simulink model "test_plant"  (R2023a)
settings: Solver=ode5  StartTime=0.0  StopTime=96  FixedStep=1.0  RelTol=1e-3
undefined symbols (not defined in the file): Standard_Devices, UDP_Protocol
libraries: sldrtlib x3, embmathops x1
settings Model: Creator=The MathWorks, Inc.  LastModifiedBy=umphaipunatipunumphai
settings SolverCC: AlgebraicLoopSolver=TrustRegion  DecoupledContinuousIntegration=on  MinimalZcImpactIntegration=on
settings DataIOCC: ReturnWorkspaceOutputs=off
settings DebuggingCC: UnconnectedInputMsg=warning  UnconnectedOutputMsg=warning  UnconnectedLineMsg=warning  PregeneratedLibrarySubsystemCodeDiagnostic=none  ArithmeticOperatorsInVariantConditions=warning
settings HardwareCC: ProdBitPerLong=64  ProdHWDeviceType=Intel->x86-64 (Linux 64)
settings ModelReferenceCC: EnableRefExpFcnMdlSchedulingChecks=on
settings SFSimCC: SimUseLocalCustomCode=off  CustomCodeUndefinedFunction=UseInterfaceOnly
settings RTWCC: Description=Simulink Desktop Real-Time  SystemTargetFile=sldrt.tlc  TemplateMakefile=sldrt.tmf  RTWUseLocalCustomCode=off  RTWCompilerOptimization=on  DLArmComputeVersion=19.05
settings CodeAppCC: MaxIdLength=95
settings SimulinkDesktopRealTimeCC: TargetLibSuffix=_sldrt.a  TargetPreCompLibLocation=/Applications/MATLAB_R2023a.app/toolbox/sldrt/lib/maci64

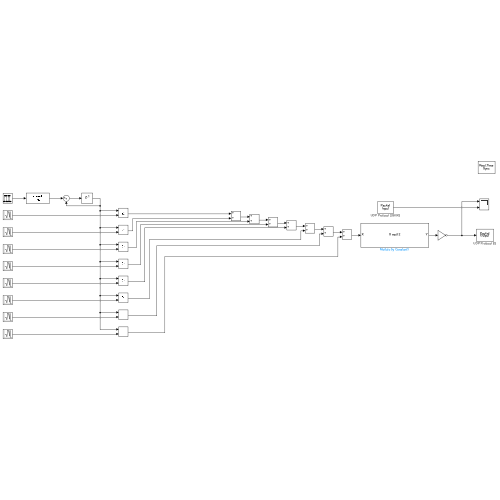
[thumbnail: Simulink's stored preview of the top-level diagram]
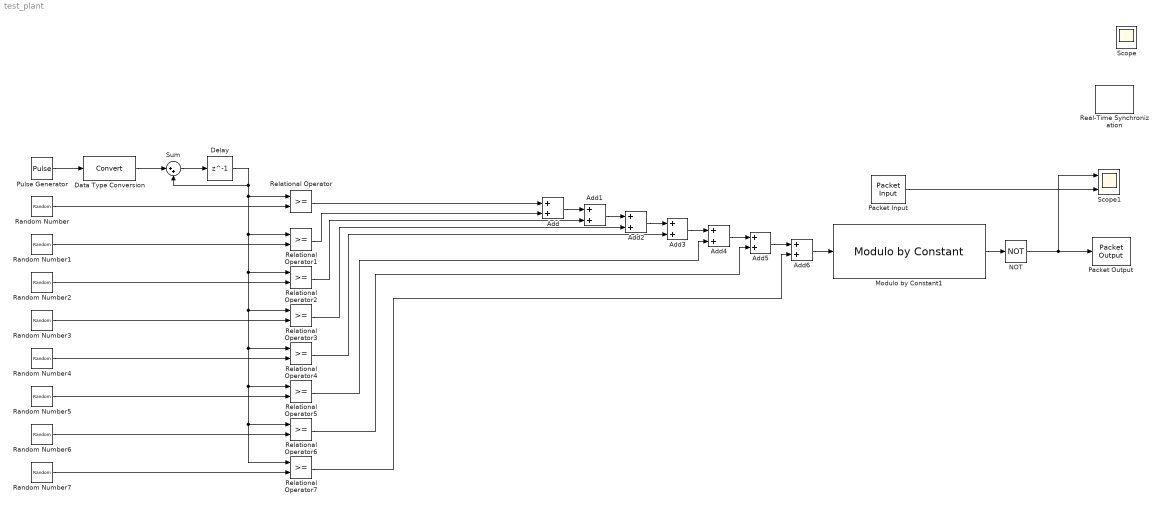
== system test_plant ==
  Add{,1..6} (7 alike) : Sum
  Data Type Conversion : DataTypeConversion  OutMin=0  OutMax=1  ConvertRealWorld=Stored Integer (SI)  RndMeth=Nearest  SaturateOnIntegerOverflow=off
  Delay : Delay  DelayLength=1  InitialCondition=0  SampleTime=1
  Modulo by Constant1 : embmathops/Modulo by Constant  Denominator=2  SimulateUsing=Code generation
      settings: LibrarySourceBlock=embeddedMathLib/Modulo by Constant
  NOT : Logic  Operator=NOT  IconShape=distinctive  AllPortsSameDT=off  OutDataTypeStr=boolean
  Packet Input : sldrtlib/Packet Input  SampleTime=1  MaxMissedTicks=10  ShowMissedTicks=off  YieldWhenWaiting=on  DrvName=Standard_Devices/UDP_Protocol  DrvAddress=26000  DrvOptions=[0 0 114 112 105 99 112 115 46 109 115 104 111 109 101 46 110 101 116 0 0 0 0 0 0 0 0 0 0 0 0 0 0 0 0 0 0 0 0 0 0 0 0 0 0 0 0 0 0 0 0 0 0 0 0 0 0 0 0 0 0 0 0 0 0 0 0 0 0 0 0 0 0 0 0 0 0 0 0 0 0 0 0 0 0 0 0 0 0 0 0 0 0 0 0 0 0 0 0 0 0 0 0 0 0 0 0 0 0 0 0 0 0 0 0 0 0 0 0 0 0 0 0 0 0 0 0 0 0 0 0 0 0 0 0 0 0 0 0 0 0 0 0 0 0 0 0 0 0 0 0 0 0 0 0 0 0 0 0 0 0 0 0 0 0 0 0 0 0 0 0 0 0 0 0 0 0 0 0 0 0 0 0 0 0 0 0 0 0 0 0 0 0 0 0 0 0 0 0 0 0 0 0 0 0 0 0 0 0 0 0 0 0 0 0 0 0 0 0 0 0 0 0 0 0 0 0 0 0 0 0 0 0 0 0 0 0 0 0 0 0 0 0 0 0 0 0 0 0 0 0 0 0 0 0 0]  PacketSize=8  DataTypes='double'  ShowReady=off  ShowError=off  PacketID=1  ByteOrder=1  ShowTimestamp=off
      settings: AttributesFormatString=UDP Protocol [26000]
  Packet Output : sldrtlib/Packet Output  SampleTime=1.0  MaxMissedTicks=10  ShowMissedTicks=off  YieldWhenWaiting=on  DrvName=Standard_Devices/UDP_Protocol  DrvAddress=0  DrvOptions=[0 25000 114 112 105 99 112 115 46 109 115 104 111 109 101 46 110 101 116 0 0 0 0 0 0 0 0 0 0 0 0 0 0 0 0 0 0 0 0 0 0 0 0 0 0 0 0 0 0 0 0 0 0 0 0 0 0 0 0 0 0 0 0 0 0 0 0 0 0 0 0 0 0 0 0 0 0 0 0 0 0 0 0 0 0 0 0 0 0 0 0 0 0 0 0 0 0 0 0 0 0 0 0 0 0 0 0 0 0 0 0 0 0 0 0 0 0 0 0 0 0 0 0 0 0 0 0 0 0 0 0 0 0 0 0 0 0 0 0 0 0 0 0 0 0 0 0 0 0 0 0 0 0 0 0 0 0 0 0 0 0 0 0 0 0 0 0 0 0 0 0 0 0 0 0 0 0 0 0 0 0 0 0 0 0 0 0 0 0 0 0 0 0 0 0 0 0 0 0 0 0 0 0 0 0 0 0 0 0 0 0 0 0 0 0 0 0 0 0 0 0 0 0 0 0 0 0 0 0 0 0 0 0 0 0 0 0 0 0 0 0 0 0 0 0 0 0 0 0 0 0 0 0 0 0 0]  PacketSize=8  DataTypes='double'  ShowReady=off  ShowError=off  PacketID=1  ByteOrder=1  InitialValue=[]  FinalValue=[]
      settings: AttributesFormatString=UDP Protocol [0]
  Pulse Generator : DiscretePulseGenerator  Period=1  SampleTime=48
  Random Number : RandomNumber  Mean=3  SampleTime=48
  Random Number1 : RandomNumber  Mean=9  Seed=1  SampleTime=48
  Random Number2 : RandomNumber  Mean=15  Seed=2  SampleTime=48
  Random Number3 : RandomNumber  Mean=21  Seed=3  SampleTime=48
  Random Number4 : RandomNumber  Mean=27  Seed=4  SampleTime=48
  Random Number5 : RandomNumber  Mean=33  Seed=5  SampleTime=48
  Random Number6 : RandomNumber  Mean=39  Seed=6  SampleTime=48
  Random Number7 : RandomNumber  Mean=45  Seed=7  SampleTime=48
  Real-Time Synchronization : sldrtlib/Real-Time Synchronization  SampleTime=1.0  MaxMissedTicks=100  ShowMissedTicks=off  YieldWhenWaiting=off
  Relational Operator{,1..7} (8 alike) : RelationalOperator  OutDataTypeStr=boolean  RndMeth=Simplest  InputSameDT=off
  Scope1 : Scope  NumInputPorts=2
  Sum : Sum  Inputs=|++
  Scope : Scope
  wires:
  Packet Input/1 -> Scope1/2
  Random Number4/1 -> Relational Operator4/2
  Random Number6/1 -> Relational Operator6/2
  Add3/1 -> Add4/1
  Modulo by Constant1/1 -> NOT/1
  Data Type Conversion/1 -> Sum/1
  Random Number7/1 -> Relational Operator7/2
  Pulse Generator/1 -> Data Type Conversion/1
  Relational Operator5/1 -> Add4/2
  Random Number3/1 -> Relational Operator3/2
  Relational Operator/1 -> Add/1
  Sum/1 -> Delay/1
  Relational Operator4/1 -> Add3/2
  Add2/1 -> Add3/1
  Delay/1 -> Relational Operator/1, Relational Operator6/1, Relational Operator7/1, Relational Operator5/1, Relational Operator4/1, Relational Operator3/1, Relational Operator2/1, Relational Operator1/1, Sum/2
  Add1/1 -> Add2/1
  Add4/1 -> Add5/1
  Add5/1 -> Add6/1
  Relational Operator2/1 -> Add1/2
  Relational Operator7/1 -> Add6/2
  Relational Operator3/1 -> Add2/2
  Add6/1 -> Modulo by Constant1/1
  Add/1 -> Add1/1
  Random Number2/1 -> Relational Operator2/2
  Relational Operator6/1 -> Add5/2
  Random Number1/1 -> Relational Operator1/2
  Random Number/1 -> Relational Operator/2
  Relational Operator1/1 -> Add/2
  Random Number5/1 -> Relational Operator5/2
  NOT/1 -> Scope1/1, Packet Output/1
